simulink model "input_test"  (R2021b)
settings: Solver=VariableStepAuto  StartTime=0.0  StopTime=25  RelTol=1e-3
values from neighbouring files (symbols this model uses):
  A = [0, 0,   1,   0 ... (first row only)    [collision_avoidance_simulation.m]
  B = [0, 0 ... (first row only)    [collision_avoidance_simulation.m]
  n_beams = 20    [collision_avoidance_simulation.m]
  Walls = [ -1,  0,  7, -3,  4 ... (first row only)    [collision_avoidance_simulation.m]
  wp = [-8, -11,  -8, 2, 12, 8, 12 ... (first row only)    [collision_avoidance_simulation.m]
libraries: vrlib x1, sldrtlib x1
settings Model: Creator=Pål  LastModifiedBy=paalhm
settings SolverCC: AlgebraicLoopSolver=TrustRegion
settings DebuggingCC: SFMachineParentedDataDiag=warning  UnderSpecifiedDimensionMsg=error

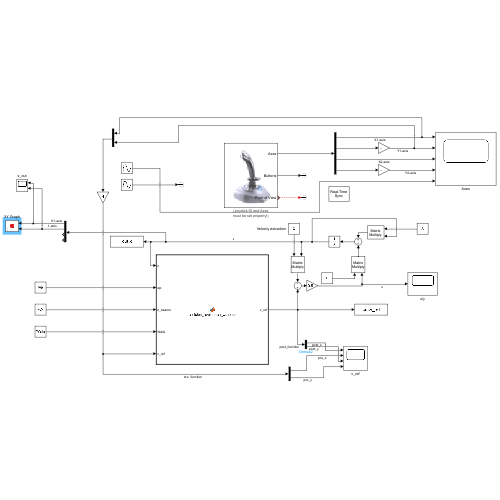
[thumbnail: Simulink's stored preview of the top-level diagram]
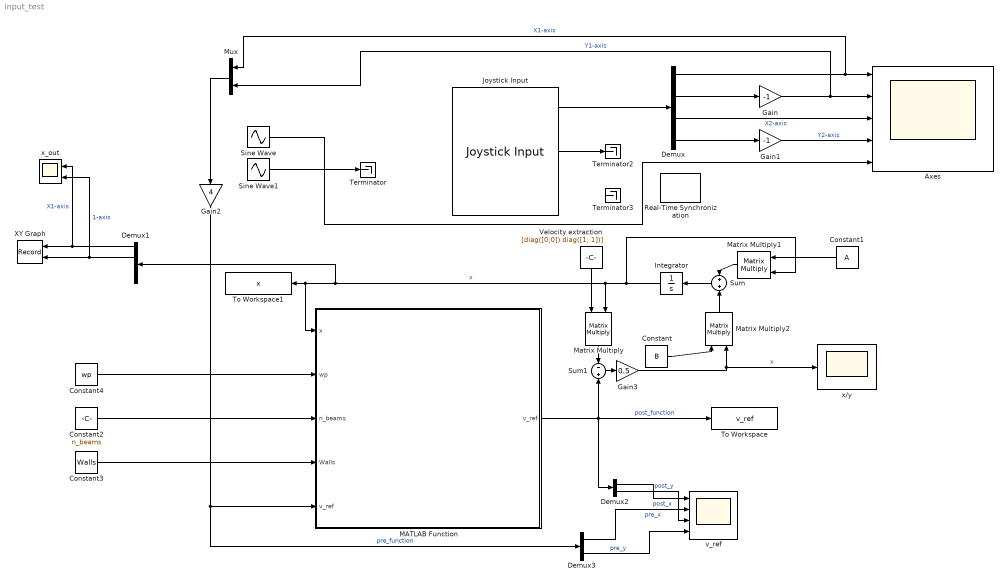
== system input_test ==
  Axes : Scope  NumInputPorts=5
  Constant : Constant  Value=B
  Constant1 : Constant  Value=A
  Constant2 : Constant  Value=n_beams
  Constant3 : Constant  Value=Walls
  Constant4 : Constant  Value=wp  VectorParams1D=off
  Demux : Demux
  Demux1 : Demux
  Demux2 : Demux  Outputs=2
  Demux3 : Demux  Outputs=2
  Gain : Gain  Gain=-1
  Gain1 : Gain  Gain=-1
  Gain2 : Gain  Gain=4
  Gain3 : Gain  Gain=0.5
  Integrator : Integrator  InitialCondition=[-9;-2;0;0]  ContinuousStateAttributes="\"x\""
  Joystick Input : vrlib/Joystick Input  joyid=1  adjustports=on  forcefeed=off
      settings: AttributesFormatString=(Joystick ID and Axes\nmust be set properly!)
  MATLAB Function : MATLAB Function  TreatAsAtomicUnit=on  SystemSampleTime=0.01
      settings: MinAlgLoopOccurrences=on
  Matrix Multiply : Product  Multiplication=Matrix(*)
  Matrix Multiply1 : Product  Multiplication=Matrix(*)
  Matrix Multiply2 : Product  Multiplication=Matrix(*)
  Mux : Mux  Inputs=2
  Real-Time Synchronization : sldrtlib/Real-Time Synchronization  SampleTime=0.1  MaxMissedTicks=200  ShowMissedTicks=off  YieldWhenWaiting=on
  Sine Wave : Sin  SampleTime=0
  Sine Wave1 : Sin  Phase=pi/2  SampleTime=0
  Sum : Sum  Inputs=+|+
  Sum1 : Sum  Inputs=-|+
  Terminator : Terminator
  Terminator2 : Terminator
  Terminator3 : Terminator
  To Workspace : ToWorkspace  VariableName=v_ref  SaveFormat=Timeseries  SampleTime=-1
  To Workspace1 : ToWorkspace  VariableName=x  SaveFormat=Timeseries  SampleTime=-1
  Velocity extraction : Constant  Value=[diag([0;0]) diag([1; 1])]
  XY Graph : Record  FileSettingsInternal="{\"entries\":[{\"content\":{\"excelSettings\":{\"content\":{},\"type\":\"Streamout.ExcelSettings\"}},\"type\":\"Streamout.FileSettingStorage\",\"uuid\":\"fa9775ad-cbb9-48f6-8807-cfcae20c46bf\"}],\"packageUris\":[\"http://schema.mathworks.com/mf0/streamout_blocks/R2020a\"],\"version\":\"1.0\"}"  Layout=[1 1]  SignalsInternal="{\"entries\":[{\"content\":{\"signals\":[{\"content\":{\"blockPath\":[\"input_test/XY Graph\"],\"channel\":[],\"dimensions\":[1],\"domain\":\"input_test/XY Graph\",\"lineColor\":\"#a2142f\",\"plots\":[],\"port\":1,\"sid\":[\"\"],\"signalID\":5444,\"signalName\":\"X1-axis\"},\"type\":\"RecordBlkView.Signal\",\"uuid\":\"8b8b7179-8c22-4817-a8d0-92590bc3d59b\"},{\"content\":{\"blockPath\":[\"input_test/XY Graph\"],\"channel\":[],\"dimensions\":[1],\"domain\":\"input_test/XY Graph\",\"lineColor\":\"#139fff\",\"plots\":[],\"port\":2,\"sid\":[\"\"],\"signalID\":5448,\"signalName\":\"1-axis\"},\"type\":\"RecordBlkView.Signal\",\"uuid\":\"4635b04d-f062-464d-b985-dbaf1a520d80\"}]},\"type\":\"RecordBlkView.InputSignals\",\"uuid\":\"af2d743c-cc46-4980-a2f8-a07ce4f3e00f\"}],\"packageUris\":[\"http://schema.mathworks.com/mf0/streamout_blocks/R2020a\"],\"version\":\"1.0\"}"  VisualizationBindings="{\"xyplotplugin\":{\"info\":[{\"series\":[],\"subplotID\":1}]}}"  CompatibilityTag=XY
  v_ref : Scope  NumInputPorts=4
  x/y : Scope
  x_out : Scope  NumInputPorts=2
  wires:
  Joystick Input/1 -> Demux/1
  Demux/1 -> Mux/1, Axes/1  "X1-axis"
  Demux/2 -> Gain/1
  Demux/3 -> Axes/3  "X2-axis"
  Demux/4 -> Gain1/1
  Gain/1 -> Mux/2, Axes/2  "Y1-axis"
  Gain1/1 -> Axes/4  "Y2-axis"
  Constant3/1 -> MATLAB Function/4(Walls)
  MATLAB Function/1(v_ref) -> Demux2/1, Sum1/2, To Workspace/1  "post_function"
  Mux/1 -> Gain2/1
  Constant4/1 -> MATLAB Function/2(wp)
  Constant2/1 -> MATLAB Function/3(n_beams)
  Joystick Input/2 -> Terminator2/1
  Integrator/1 -> Matrix Multiply1/2, Matrix Multiply/2, Demux1/1, To Workspace1/1, MATLAB Function/1(x)  "x"
  ? -> Terminator3/1
  Sine Wave/1 -> Axes/5
  Matrix Multiply/1 -> Sum1/1
  Sum/1 -> Integrator/1
  Matrix Multiply1/1 -> Sum/1
  Matrix Multiply2/1 -> Sum/2
  Velocity extraction/1 -> Matrix Multiply/1
  Constant/1 -> Matrix Multiply2/1
  Constant1/1 -> Matrix Multiply1/1
  Gain2/1 -> Demux3/1, MATLAB Function/5("v_ref ")  "pre_function"
  Demux1/1 -> XY Graph/1, x_out/1  "X1-axis"
  Demux1/2 -> XY Graph/2, x_out/2  "1-axis"
  Sum1/1 -> Gain3/1
  Gain3/1 -> x/y/1, Matrix Multiply2/2  "x"
  Sine Wave1/1 -> Terminator/1
  Demux2/1 -> v_ref/1  "post_x"
  Demux2/2 -> v_ref/3  "post_y"
  Demux3/1 -> v_ref/2  "pre_x"
  Demux3/2 -> v_ref/4  "pre_y"

== matlab function input_test/MATLAB Function ==
  data: x input; v_ref output; wp input; n_beams input; Walls input; v_ref input
function v_ref = collision_avoidance_wrapper(x, wp, n_beams, Walls, v_ref)
function v_ref = collision_avoidance_wrapper(x, wp, n_beams, Walls, v_ref)
    persistent w

    if isempty(w)
        w = 1;
    end
    [points, ranges, ~] = findAllRange(x(1:2),n_beams,Walls);
    beams = [points-x(1:2);ranges'];
    v_ref = collision_avoidance(beams, x, 1, 2, v_ref, 4);
    
%     if norm(x(1:2)-wp(:,round(w))) < 0.5
%         w = w + 1;
%         if w == length(wp)+1
%             w = -1;
%             return
%         end
%         plot(wp(1,w),wp(2,w), 'r*')
%     end
end
